simulink model "pendulumExample2"  (Simulink 7.3)
settings: Solver=ode3  StartTime=0.0  StopTime=tof  FixedStep=0.01  RelTol=1e-3
InitFcn:
  | initPendulum2
StopFcn:
  | plotlab
values from neighbouring files (symbols this model uses):
  Arm = [0 1;-wn^2 -2*ksi*wn]    [init.m]    (also in initPendulum2.m)
  B = [0 1]'    [init.m]    (also in initPendulum2.m = [0 0 ; 0 1])
  Brm = [0 wn^2]'    [init.m]    (also in initPendulum2.m)
  epsilon = 0.08    [init.m]    (also in initPendulum2.m)
  GammaW = 3.5    [init.m]    (also in initPendulum2.m)
  K = [1.5 0;0 1.3]    [init.m]    (also in initPendulum2.m)
  nofbasis = 3    [initPendulum2.m]
  nofstates = 2    [initPendulum2.m]
  P = lyap(A',Q)    [init.m]    (also in initPendulum2.m)
  pMax = 10    [initPendulum2.m]
  W0 = [2 -0.5 1]'    [init.m]    (also in initPendulum2.m = [2 -0.5 1 ; 0 0 0]')
  x0 = [1 1]'    [init.m]    (also in initPendulum2.m)
libraries: dspbuff3 x2, simulink x1, dspmtrx3 x1
settings Model: Creator=Alp  LastModifiedBy=alp.marangoz

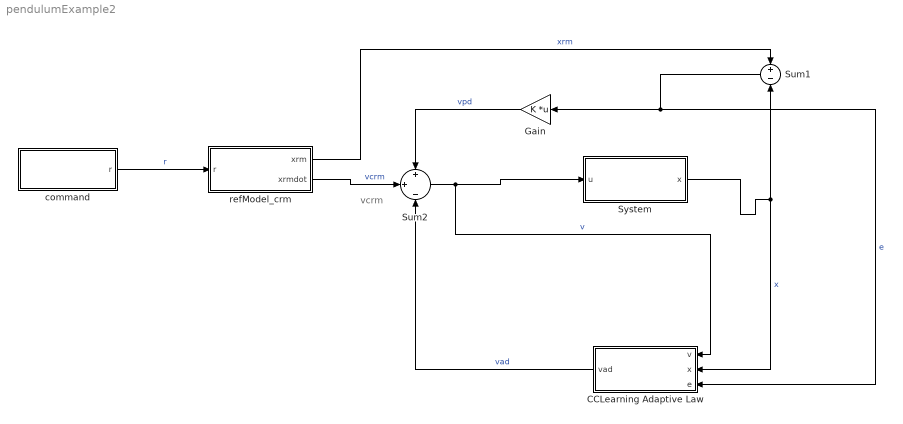
== system pendulumExample2 ==
  note: vcrm
  CCLearning Adaptive Law : Subsystem  TreatAsAtomicUnit=on
  Gain : Gain  Gain=K  Multiplication=Matrix(K*u)  ParameterDataType=fixdt(1, 16)  ParameterScaling=2^0  OutDataType=fixdt(1, 16)  OutScaling=2^0
  Sum1 : Sum  Inputs=+|-  OutDataType=fixdt(1, 16)  OutScaling=2^0
  Sum2 : Sum  Inputs=+|+|-  OutDataType=fixdt(1, 16)  OutScaling=2^0
  System : Subsystem  TreatAsAtomicUnit=on
  command : Subsystem
  refModel_crm : Subsystem  TreatAsAtomicUnit=on
  wires:
  command/1(r) -> refModel_crm/1(r)  "r"
  refModel_crm/1(xrm) -> Sum1/1  "xrm"
  Sum1/1 -> Gain/1, CCLearning Adaptive Law/3(e)  "e"
  Gain/1 -> Sum2/1  "vpd"
  refModel_crm/2(xrmdot) -> Sum2/2  "vcrm"
  Sum2/1 -> System/1(u), CCLearning Adaptive Law/1(v)  "v"
  CCLearning Adaptive Law/1(vad) -> Sum2/3  "vad"
  System/1(x) -> Sum1/2, CCLearning Adaptive Law/2(x)  "x"

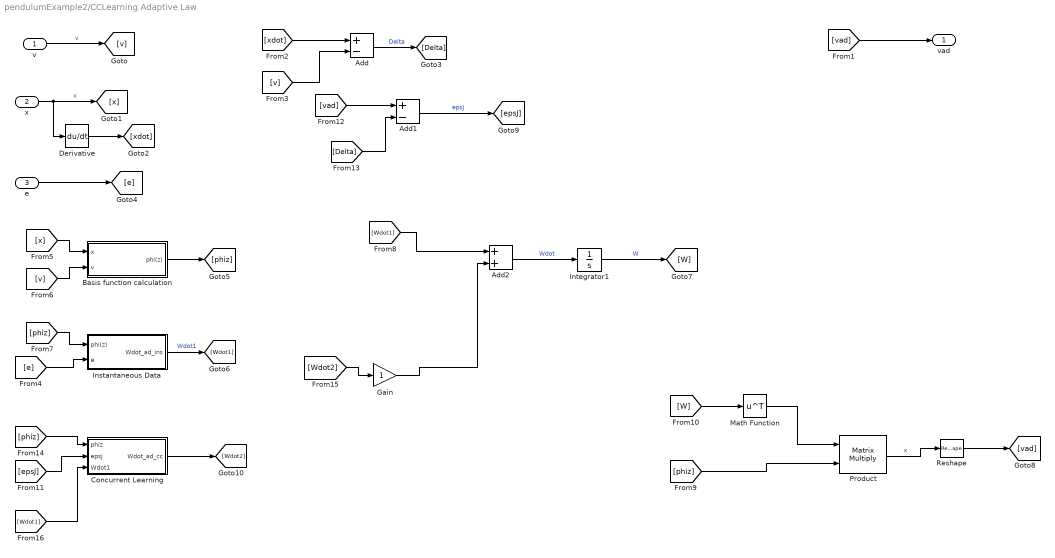
== system pendulumExample2/CCLearning Adaptive Law ==
  v : Inport  OutDataType=fixdt(1, 16)  OutScaling=2^0
  x : Inport  Port=2  OutDataType=fixdt(1, 16)  OutScaling=2^0
  e : Inport  Port=3  OutDataType=fixdt(1, 16)  OutScaling=2^0
  Add : Sum  Inputs=+-  OutDataType=fixdt(1, 16)  OutScaling=2^-10
  Add1 : Sum  Inputs=+-  OutDataType=fixdt(1, 16)  OutScaling=2^-10
  Add2 : Sum  OutDataType=fixdt(1, 16)  OutScaling=2^-10
  Basis function calculation : Subsystem  TreatAsAtomicUnit=on
  Concurrent Learning : Subsystem  TreatAsAtomicUnit=on
  Derivative : Derivative
  Gain : Gain  ParameterDataType=fixdt(1, 16)  ParameterScaling=2^0  OutDataType=fixdt(1, 16)  OutScaling=2^0
  Instantaneous Data : Subsystem  TreatAsAtomicUnit=on
  Integrator1 : Integrator  InitialCondition=W0
  Math Function : Math  Operator=transpose  OutDataType=fixdt(1, 16)  OutScaling=2^0  SaturateOnIntegerOverflow=on
  Product : Product  Multiplication=Matrix(*)  OutDataType=fixdt(1, 16)  OutScaling=2^0  RndMeth=Zero
  Reshape : Reshape  OutputDimensionality=Column vector (2-D)
  vad : Outport  OutDataType=fixdt(1, 16)  OutScaling=2^0
  wires:
  v/1 -> [v]  "v"
  [vad] -> vad/1
  x/1 -> [x], Derivative/1  "x"
  Derivative/1 -> [xdot]
  [xdot] -> Add/1
  [v] -> Add/2
  Add/1 -> [Delta]  "Delta"
  e/1 -> [e]
  [e] -> Instantaneous Data/2(e)
  [x] -> Basis function calculation/1(x)
  [v] -> Basis function calculation/2(v)
  Basis function calculation/1(phi(z)) -> [phiz]
  [phiz] -> Instantaneous Data/1(phi(z))
  Instantaneous Data/1(Wdot_ad_ins) -> [Wdot1]  "Wdot1"
  Integrator1/1 -> [W]  "W"
  [W] -> Math Function/1
  Math Function/1 -> Product/1
  [phiz] -> Product/2
  Product/1 -> Reshape/1  "x"
  Reshape/1 -> [vad]
  [vad] -> Add1/1
  [Delta] -> Add1/2
  Add1/1 -> [epsJ]  "epsJ"
  [phiz] -> Concurrent Learning/1(phiz)
  Concurrent Learning/1(Wdot_ad_cc) -> [Wdot2]
  [epsJ] -> Concurrent Learning/2(epsj)
  [Wdot1] -> Add2/1
  Add2/1 -> Integrator1/1  "Wdot"
  [Wdot2] -> Gain/1
  [Wdot1] -> Concurrent Learning/3(Wdot1)
  Gain/1 -> Add2/2

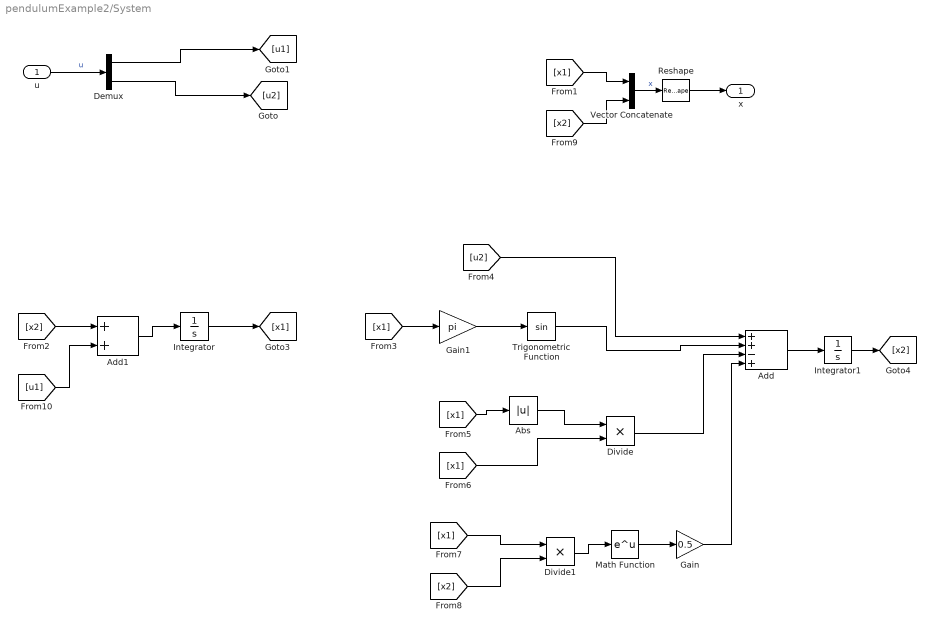
== system pendulumExample2/System ==
  u : Inport  OutDataType=fixdt(1, 16)  OutScaling=2^0
  Abs : Abs  OutDataType=fixdt(1, 16)  OutScaling=2^0
  Add : Sum  Inputs=++-+  OutDataType=fixdt(1, 16)  OutScaling=2^-10
  Add1 : Sum  OutDataType=fixdt(1, 16)  OutScaling=2^-10
  Demux : Demux  Outputs=2
  Divide : Product  Inputs=**  OutDataType=fixdt(1, 16)  OutScaling=2^-10
  Divide1 : Product  Inputs=**  OutDataType=fixdt(1, 16)  OutScaling=2^-10
  Gain : Gain  Gain=0.5  ParameterDataType=fixdt(1, 16)  ParameterScaling=2^0  OutDataType=fixdt(1, 16)  OutScaling=2^0
  Gain1 : Gain  Gain=pi  ParameterDataType=fixdt(1, 16)  ParameterScaling=2^0  OutDataType=fixdt(1, 16)  OutScaling=2^0
  Integrator : Integrator  InitialCondition=x0(1,1)
  Integrator1 : Integrator  InitialCondition=x0(2,1)
  Math Function : Math  OutDataType=fixdt(1, 16)  OutScaling=2^0  SaturateOnIntegerOverflow=on
  Reshape : Reshape  OutputDimensionality=Column vector (2-D)
  Trigonometric Function : Trigonometry
  Vector Concatenate : Concatenate  Mode=Vector
  x : Outport  OutDataType=fixdt(1, 16)  OutScaling=2^0
  wires:
  Integrator/1 -> [x1]
  [x1] -> Gain1/1
  [x1] -> Abs/1
  Abs/1 -> Divide/1
  [x1] -> Divide/2
  [x1] -> Divide1/1
  [x2] -> Divide1/2
  Divide1/1 -> Math Function/1
  Math Function/1 -> Gain/1
  [u2] -> Add/1
  Trigonometric Function/1 -> Add/2
  Divide/1 -> Add/3
  Gain/1 -> Add/4
  Add/1 -> Integrator1/1
  Integrator1/1 -> [x2]
  [x1] -> Vector Concatenate/1
  [x2] -> Vector Concatenate/2
  Vector Concatenate/1 -> Reshape/1  "x"
  Reshape/1 -> x/1
  u/1 -> Demux/1  "u"
  Demux/1 -> [u1]
  Demux/2 -> [u2]
  Gain1/1 -> Trigonometric Function/1
  [x2] -> Add1/1
  Add1/1 -> Integrator/1
  [u1] -> Add1/2

== system pendulumExample2/command ==
  Demux : Demux  Outputs=2
  From Workspace : FromWorkspace  VariableName=rData  OutputAfterFinalValue=Setting to zero
  Reshape : Reshape  OutputDimensionality=Column vector (2-D)
  Terminator1 : Terminator
  r : Outport
  wires:
  From Workspace/1 -> Reshape/1  "r"
  Reshape/1 -> Demux/1
  Demux/1 -> Terminator1/1  "r1"
  Demux/2 -> r/1  "r2"

== system pendulumExample2/refModel_crm ==
  r : Inport  OutDataType=fixdt(1, 16)  OutScaling=2^0
  Add1 : Sum  OutDataType=fixdt(1, 16)  OutScaling=2^-10
  Gain1 : Gain  Gain=Arm  Multiplication=Matrix(K*u)  ParameterDataType=fixdt(1, 16)  ParameterScaling=2^0  OutDataType=fixdt(1, 16)  OutScaling=2^0
  Gain2 : Gain  Gain=Brm  Multiplication=Matrix(K*u)  ParameterDataType=fixdt(1, 16)  ParameterScaling=2^0  OutDataType=fixdt(1, 16)  OutScaling=2^0
  Integrator : Integrator  InitialCondition=x0
  Reshape : Reshape  OutputDimensionality=Column vector (2-D)
  xrm : Outport  OutDataType=fixdt(1, 16)  OutScaling=2^0
  xrmdot : Outport  Port=2  OutDataType=fixdt(1, 16)  OutScaling=2^0
  wires:
  [x] -> Gain1/1
  r/1 -> [u]  "r"
  [u] -> Gain2/1
  Gain1/1 -> Add1/1
  Gain2/1 -> Add1/2
  Add1/1 -> Reshape/1  "xrmdot"
  Integrator/1 -> xrm/1, [x]  "xrm"
  Reshape/1 -> Integrator/1, xrmdot/1

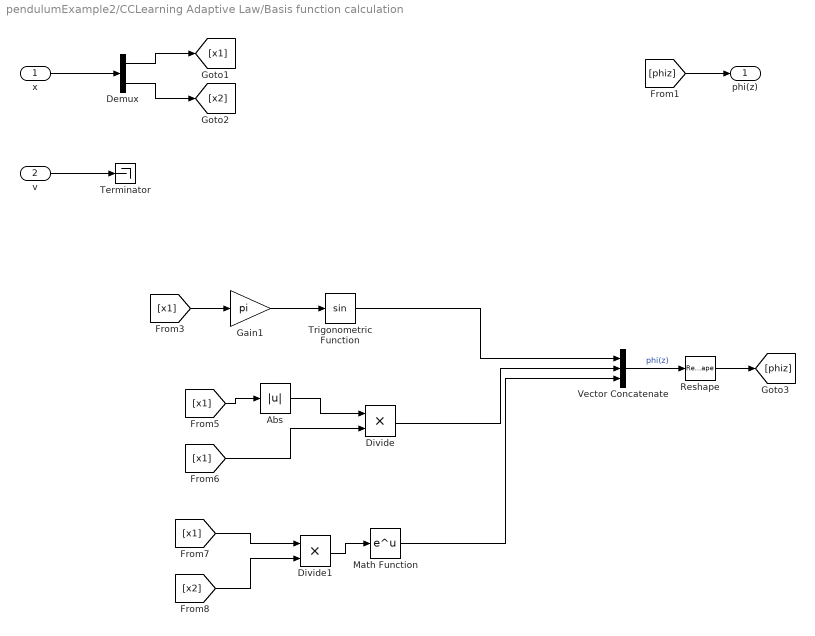
== system pendulumExample2/CCLearning Adaptive Law/Basis function calculation ==
  x : Inport  OutDataType=fixdt(1, 16)  OutScaling=2^0
  v : Inport  Port=2  OutDataType=fixdt(1, 16)  OutScaling=2^0
  Abs : Abs  OutDataType=fixdt(1, 16)  OutScaling=2^0
  Demux : Demux  Outputs=2
  Divide : Product  Inputs=**  OutDataType=fixdt(1, 16)  OutScaling=2^-10
  Divide1 : Product  Inputs=**  OutDataType=fixdt(1, 16)  OutScaling=2^-10
  Gain1 : Gain  Gain=pi  ParameterDataType=fixdt(1, 16)  ParameterScaling=2^0  OutDataType=fixdt(1, 16)  OutScaling=2^0
  Math Function : Math  OutDataType=fixdt(1, 16)  OutScaling=2^0  SaturateOnIntegerOverflow=on
  Reshape : Reshape  OutputDimensionality=Column vector (2-D)
  Terminator : Terminator
  Trigonometric Function : Trigonometry
  Vector Concatenate : Concatenate  NumInputs=3  Mode=Vector
  phi(z) : Outport  OutDataType=fixdt(1, 16)  OutScaling=2^0
  wires:
  x/1 -> Demux/1
  v/1 -> Terminator/1
  [phiz] -> phi(z)/1
  [x1] -> Gain1/1
  [x1] -> Abs/1
  Abs/1 -> Divide/1
  [x1] -> Divide/2
  [x1] -> Divide1/1
  [x2] -> Divide1/2
  Divide1/1 -> Math Function/1
  Gain1/1 -> Trigonometric Function/1
  Demux/1 -> [x1]
  Demux/2 -> [x2]
  Vector Concatenate/1 -> Reshape/1  "phi(z)"
  Reshape/1 -> [phiz]
  Trigonometric Function/1 -> Vector Concatenate/1
  Divide/1 -> Vector Concatenate/2
  Math Function/1 -> Vector Concatenate/3

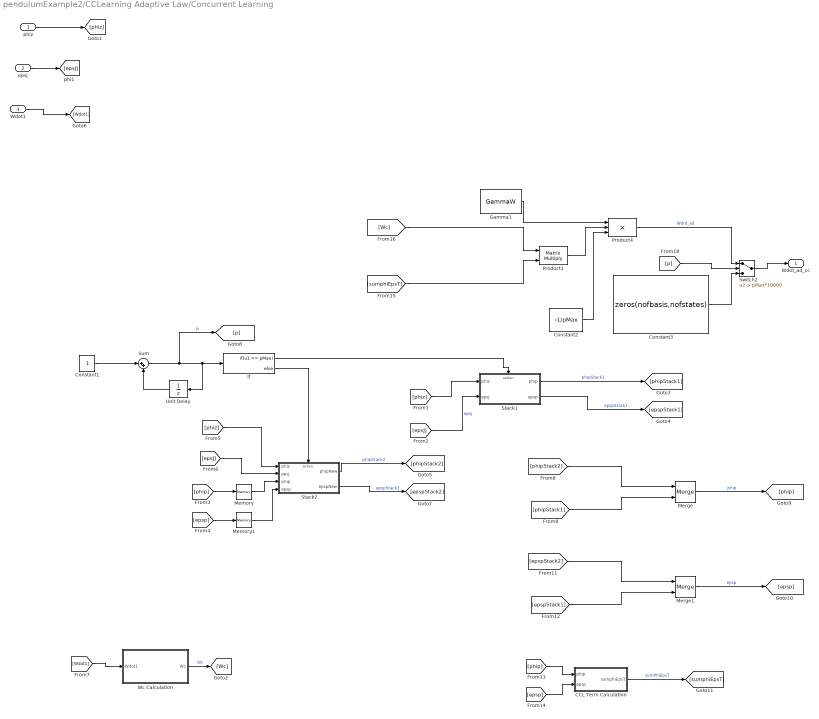
== system pendulumExample2/CCLearning Adaptive Law/Concurrent Learning ==
  phiz : Inport  OutDataType=fixdt(1, 16)  OutScaling=2^0
  epsj : Inport  Port=2  OutDataType=fixdt(1, 16)  OutScaling=2^0
  Wdot1 : Inport  Port=3
  CCL Term Calculation : Subsystem  TreatAsAtomicUnit=on
  Constant1 : Constant  OutDataType=fixdt(1, 16)  OutScaling=2^0  SampleTime=-1
  Constant2 : Constant  Value=-1/pMax  OutDataType=fixdt(1, 16)  OutScaling=2^0
  Constant3 : Constant  Value=zeros(nofbasis,nofstates)  OutDataType=fixdt(1, 16)  OutScaling=2^0  SampleTime=-1
  Gamma1 : Constant  Value=GammaW  VectorParams1D=off  OutDataType=fixdt(1, 16)  OutScaling=2^0
  If : If  IfExpression=u1 <= pMax
  Memory : Memory  X0=zeros(nofbasis,pMax)  InheritSampleTime=on  LinearizeMemory=on  LinearizeAsDelay=on
  Memory1 : Memory  X0=zeros(nofstates,pMax)  InheritSampleTime=on  LinearizeMemory=on  LinearizeAsDelay=on
  Merge : Merge
  Merge1 : Merge
  Product1 : Product  Multiplication=Matrix(*)  OutDataType=fixdt(1, 16)  OutScaling=2^0  RndMeth=Zero
  Product4 : Product  Inputs=3  OutDataType=fixdt(1, 16)  OutScaling=2^0  RndMeth=Zero
  Stack1 : Subsystem  TreatAsAtomicUnit=on
  Stack2 : Subsystem  TreatAsAtomicUnit=on
  Sum : Sum  Inputs=|++  OutDataType=fixdt(1, 16)  OutScaling=2^0
  Switch2 : Switch  Criteria=u2 > Threshold  Threshold=pMax*10000  OutDataType=fixdt(1, 16)  OutScaling=2^0
  Unit Delay : UnitDelay  SampleTime=-1
  Wc Calculation : Subsystem
  Wdot_ad_cc : Outport  OutDataType=fixdt(1, 16)  OutScaling=2^0
  wires:
  phiz/1 -> [phiz]
  epsj/1 -> [epsJ]
  Wdot1/1 -> [Wdot1]
  Gamma1/1 -> Product4/1
  Constant1/1 -> Sum/1
  Sum/1 -> Unit Delay/1, If/1, [p]  "p"
  Unit Delay/1 -> Sum/2
  If/1 -> Stack1/Action
  [epsJ] -> Stack1/2(epsj)  "epsj"
  Stack1/1(phip) -> [phipStack1]  "phipStack1"
  Stack1/2(epsp) -> [epspStack1]  "epspStack1"
  [phiz] -> Stack2/1(phiz)
  [epsJ] -> Stack2/2(epsj)
  If/2 -> Stack2/Action
  [phip] -> Memory/1
  Memory/1 -> Stack2/3(phip)
  [epsp] -> Memory1/1
  Memory1/1 -> Stack2/4(epsp)
  Stack2/1(phipNew) -> [phipStack2]  "phipStack2"
  Stack2/2(epspNew) -> [epspStack2]  "epspStack2"
  [phiz] -> Stack1/1(phiz)
  Merge/1 -> [phip]  "phip"
  Merge1/1 -> [epsp]  "epsp"
  [phip] -> CCL Term Calculation/1(phip)
  [epsp] -> CCL Term Calculation/2(epsp)
  CCL Term Calculation/1(sumphiEpsT) -> [sumphiEpsT]  "sumPhiEpsT"
  Constant2/1 -> Product4/3
  [Wc] -> Product1/1
  [sumphiEpsT] -> Product1/2
  Product1/1 -> Product4/2
  [p] -> Switch2/2
  Constant3/1 -> Switch2/3
  Product4/1 -> Switch2/1  "Wdot_ad"
  Switch2/1 -> Wdot_ad_cc/1
  [phipStack2] -> Merge/1
  [phipStack1] -> Merge/2
  [epspStack2] -> Merge1/1
  [epspStack1] -> Merge1/2
  [Wdot1] -> Wc Calculation/1(Wdot1)
  Wc Calculation/1(Wc) -> [Wc]  "Wc"

== system pendulumExample2/CCLearning Adaptive Law/Instantaneous Data ==
  phi(z) : Inport  OutDataType=fixdt(1, 16)  OutScaling=2^0
  e : Inport  Port=2  OutDataType=fixdt(1, 16)  OutScaling=2^0
  Gain : Gain  Gain=-1  ParameterDataType=fixdt(1, 16)  ParameterScaling=2^0  OutDataType=fixdt(1, 16)  OutScaling=2^0
  Gamma : Constant  Value=GammaW  VectorParams1D=off  OutDataType=fixdt(1, 16)  OutScaling=2^0
  P : Constant  Value=P  VectorParams1D=off  OutDataType=fixdt(1, 16)  OutScaling=2^0
  Product1 : Product  Multiplication=Matrix(*)  OutDataType=fixdt(1, 16)  OutScaling=2^0  RndMeth=Zero
  Product2 : Product  OutDataType=fixdt(1, 16)  OutScaling=2^0  RndMeth=Zero
  Product3 : Product  Multiplication=Matrix(*)  OutDataType=fixdt(1, 16)  OutScaling=2^0  RndMeth=Zero
  Product5 : Product  Multiplication=Matrix(*)  OutDataType=fixdt(1, 16)  OutScaling=2^0  RndMeth=Zero
  Transpose2 : dspmtrx3/Transpose  SystemSampleTime=-1  Hermitian=off  overflowFlag=off
  b : Constant  Value=B  VectorParams1D=off  OutDataType=fixdt(1, 16)  OutScaling=2^0
  Wdot_ad_ins : Outport  OutDataType=fixdt(1, 16)  OutScaling=2^0
  wires:
  P/1 -> Product5/1
  b/1 -> Product5/2
  e/1 -> Transpose2/1
  Transpose2/1 -> Product1/1
  Product5/1 -> Product1/2
  phi(z)/1 -> Product3/1
  Product1/1 -> Product3/2
  Gamma/1 -> Product2/1
  Product3/1 -> Product2/2
  Product2/1 -> Gain/1
  Gain/1 -> Wdot_ad_ins/1

== system pendulumExample2/CCLearning Adaptive Law/Concurrent Learning/CCL Term Calculation ==
  phip : Inport  OutDataType=fixdt(1, 16)  OutScaling=2^0
  epsp : Inport  Port=2  OutDataType=fixdt(1, 16)  OutScaling=2^0
  For Iterator Subsystem : Subsystem  TreatAsAtomicUnit=on
  Memory2 : Memory  X0=zeros(size(W0))  InheritSampleTime=on  LinearizeMemory=on  LinearizeAsDelay=on
  sumphiEpsT : Outport  OutDataType=fixdt(1, 16)  OutScaling=2^0
  wires:
  epsp/1 -> [epsp]
  phip/1 -> [phip]
  [phip] -> For Iterator Subsystem/1(phip)
  [epsp] -> For Iterator Subsystem/2(epsp)
  For Iterator Subsystem/2(forSumphiEpsTnext) -> Memory2/1
  Memory2/1 -> For Iterator Subsystem/3(forSumphiEpsT)
  For Iterator Subsystem/1(sumphiEpsT) -> [sumphiEpsT]
  [sumphiEpsT] -> sumphiEpsT/1

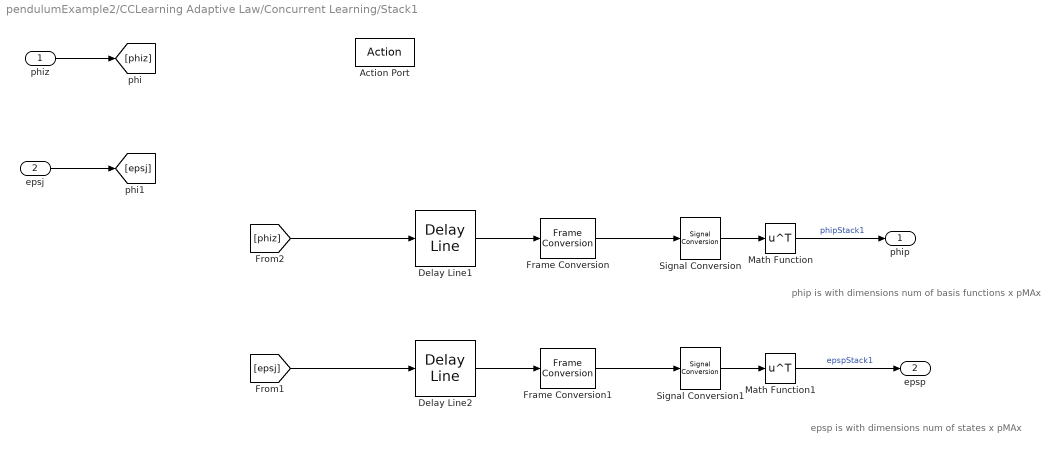
== system pendulumExample2/CCLearning Adaptive Law/Concurrent Learning/Stack1 ==
  note: phip is with dimensions num of basis functions x pMAx
  note: epsp is with dimensions num of states x pMAx
  phiz : Inport  OutDataType=fixdt(1, 16)  OutScaling=2^0
  epsj : Inport  Port=2  OutDataType=fixdt(1, 16)  OutScaling=2^0
  Action Port : ActionPort  ActionType=then
  Delay Line1 : dspbuff3/Delay Line  siz=pMax  ic=0  directfeed=on  enable_output=off  hold_output=off
  Delay Line2 : dspbuff3/Delay Line  siz=pMax  ic=0  directfeed=on  enable_output=off  hold_output=off
  Frame Conversion : FrameConversion  OutFrame=Sample-based
  Frame Conversion1 : FrameConversion  OutFrame=Sample-based
  Math Function : Math  Operator=transpose  OutDataType=fixdt(1, 16)  OutScaling=2^0  SaturateOnIntegerOverflow=on
  Math Function1 : Math  Operator=transpose  OutDataType=fixdt(1, 16)  OutScaling=2^0  SaturateOnIntegerOverflow=on
  Signal Conversion : SignalConversion  ConversionOutput=Contiguous copy
  Signal Conversion1 : SignalConversion  ConversionOutput=Contiguous copy
  phip : Outport  OutDataType=fixdt(1, 16)  OutScaling=2^0
  epsp : Outport  Port=2  OutDataType=fixdt(1, 16)  OutScaling=2^0
  wires:
  phiz/1 -> [phiz]
  Delay Line1/1 -> Frame Conversion/1
  epsj/1 -> [epsj]
  Frame Conversion/1 -> Signal Conversion/1
  [phiz] -> Delay Line1/1
  Delay Line2/1 -> Frame Conversion1/1
  Frame Conversion1/1 -> Signal Conversion1/1
  [epsj] -> Delay Line2/1
  Signal Conversion/1 -> Math Function/1
  Signal Conversion1/1 -> Math Function1/1
  Math Function/1 -> phip/1  "phipStack1"
  Math Function1/1 -> epsp/1  "epspStack1"

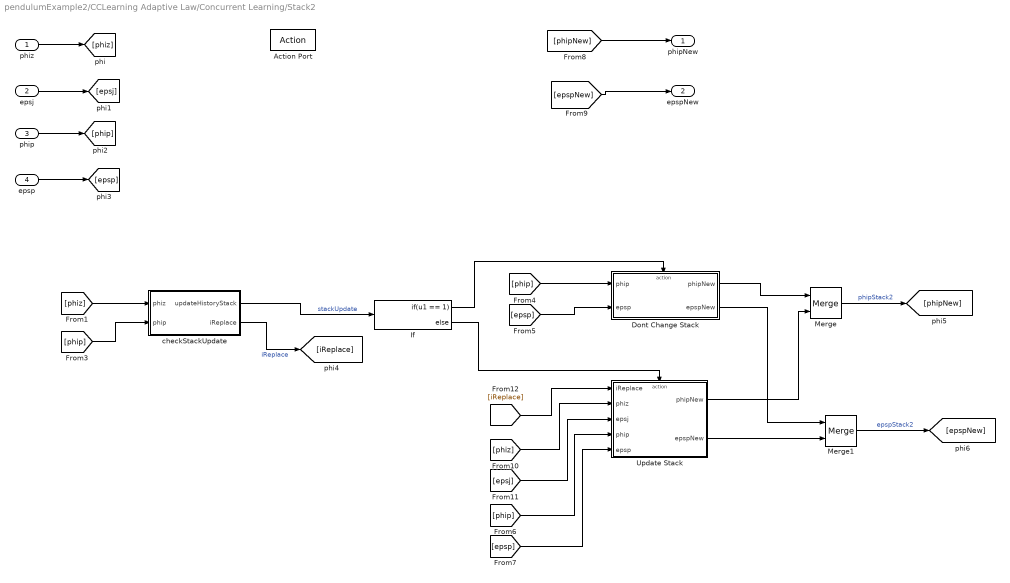
== system pendulumExample2/CCLearning Adaptive Law/Concurrent Learning/Stack2 ==
  phiz : Inport  OutDataType=fixdt(1, 16)  OutScaling=2^0
  epsj : Inport  Port=2  OutDataType=fixdt(1, 16)  OutScaling=2^0
  phip : Inport  Port=3  OutDataType=fixdt(1, 16)  OutScaling=2^0
  epsp : Inport  Port=4  OutDataType=fixdt(1, 16)  OutScaling=2^0
  Action Port : ActionPort  ActionType=else
  Dont Change Stack : Subsystem  TreatAsAtomicUnit=on
  If : If  IfExpression=u1 == 1
  Merge : Merge
  Merge1 : Merge
  Update Stack : Subsystem  TreatAsAtomicUnit=on
  checkStackUpdate : Subsystem  TreatAsAtomicUnit=on
  phipNew : Outport  OutDataType=fixdt(1, 16)  OutScaling=2^0
  epspNew : Outport  Port=2  OutDataType=fixdt(1, 16)  OutScaling=2^0
  wires:
  epsj/1 -> [epsj]
  phiz/1 -> [phiz]
  epsp/1 -> [epsp]
  phip/1 -> [phip]
  [phipNew] -> phipNew/1
  [epspNew] -> epspNew/1
  If/1 -> Dont Change Stack/Action
  If/2 -> Update Stack/Action
  [iReplace] -> Update Stack/1(iReplace)
  [phiz] -> Update Stack/2(phiz)
  [epsj] -> Update Stack/3(epsj)
  [phip] -> Update Stack/4(phip)
  [epsp] -> Update Stack/5(epsp)
  Dont Change Stack/1(phipNew) -> Merge/1
  Dont Change Stack/2(epspNew) -> Merge1/1
  Update Stack/1(phipNew) -> Merge/2
  Update Stack/2(epspNew) -> Merge1/2
  [phip] -> Dont Change Stack/1(phip)
  [epsp] -> Dont Change Stack/2(epsp)
  Merge/1 -> [phipNew]  "phipStack2"
  Merge1/1 -> [epspNew]  "epspStack2"
  [phiz] -> checkStackUpdate/1(phiz)
  [phip] -> checkStackUpdate/2(phip)
  checkStackUpdate/1(updateHistoryStack) -> If/1  "stackUpdate"
  checkStackUpdate/2(iReplace) -> [iReplace]  "iReplace"

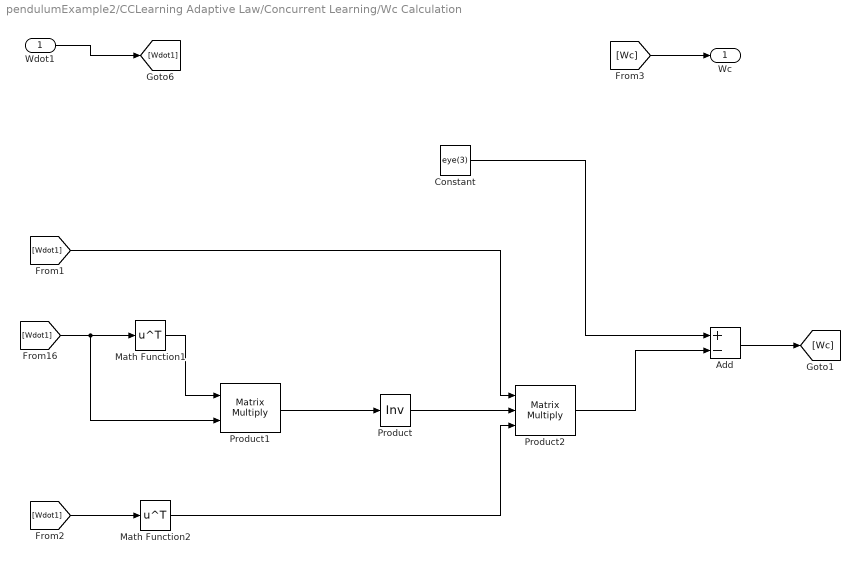
== system pendulumExample2/CCLearning Adaptive Law/Concurrent Learning/Wc Calculation ==
  Wdot1 : Inport
  Add : Sum  Inputs=+-  OutDataType=fixdt(1, 16)  OutScaling=2^-10
  Constant : Constant  Value=eye(3)  OutDataType=fixdt(1, 16)  OutScaling=2^0
  Math Function1 : Math  Operator=transpose  OutDataType=fixdt(1, 16)  OutScaling=2^0  SaturateOnIntegerOverflow=on
  Math Function2 : Math  Operator=transpose  OutDataType=fixdt(1, 16)  OutScaling=2^0  SaturateOnIntegerOverflow=on
  Product : Product  Inputs=/  Multiplication=Matrix(*)  OutDataType=fixdt(1, 16)  OutScaling=2^0  RndMeth=Zero
  Product1 : Product  Multiplication=Matrix(*)  OutDataType=fixdt(1, 16)  OutScaling=2^0  RndMeth=Zero
  Product2 : Product  Inputs=***  Multiplication=Matrix(*)  OutDataType=fixdt(1, 16)  OutScaling=2^0  RndMeth=Zero
  Wc : Outport
  wires:
  [Wdot1] -> Math Function1/1, Product1/2
  Math Function1/1 -> Product1/1
  Product1/1 -> Product/1
  Wdot1/1 -> [Wdot1]
  [Wdot1] -> Math Function2/1
  [Wdot1] -> Product2/1
  Product/1 -> Product2/2
  Math Function2/1 -> Product2/3
  Constant/1 -> Add/1
  Add/1 -> [Wc]
  [Wc] -> Wc/1
  Product2/1 -> Add/2

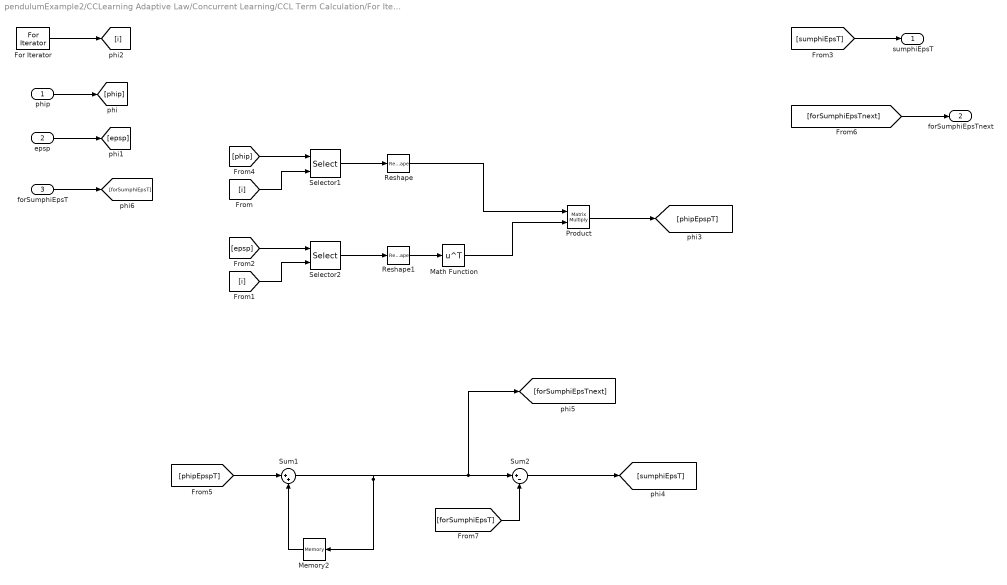
== system pendulumExample2/CCLearning Adaptive Law/Concurrent Learning/CCL Term Calculation/For Iterator Subsystem ==
  phip : Inport  OutDataType=fixdt(1, 16)  OutScaling=2^0
  epsp : Inport  Port=2  OutDataType=fixdt(1, 16)  OutScaling=2^0
  forSumphiEpsT : Inport  Port=3  OutDataType=fixdt(1, 16)  OutScaling=2^0
  For Iterator : ForIterator  IterationLimit=pMax
  Math Function : Math  Operator=transpose  OutDataType=fixdt(1, 16)  OutScaling=2^0  SaturateOnIntegerOverflow=on
  Memory2 : Memory  X0=zeros(size(W0))  InheritSampleTime=on  LinearizeMemory=on  LinearizeAsDelay=on
  Product : Product  Multiplication=Matrix(*)  OutDataType=fixdt(1, 16)  OutScaling=2^0  RndMeth=Zero
  Reshape : Reshape  OutputDimensionality=Column vector (2-D)
  Reshape1 : Reshape  OutputDimensionality=Column vector (2-D)
  Selector1 : Selector  NumberOfDimensions=2  InputPortWidth=3  IndexOptions=Select all,Index vector (port)  Indices=[1 2 3],1  OutputSizes=1,1
  Selector2 : Selector  NumberOfDimensions=2  InputPortWidth=3  IndexOptions=Select all,Index vector (port)  Indices=[1 2 3],1  OutputSizes=1,1
  Sum1 : Sum  Inputs=|++  OutDataType=fixdt(1, 16)  OutScaling=2^0
  Sum2 : Sum  Inputs=|+-  OutDataType=fixdt(1, 16)  OutScaling=2^0
  sumphiEpsT : Outport  OutDataType=fixdt(1, 16)  OutScaling=2^0
  forSumphiEpsTnext : Outport  Port=2  OutDataType=fixdt(1, 16)  OutScaling=2^0
  wires:
  epsp/1 -> [epsp]
  phip/1 -> [phip]
  For Iterator/1 -> [i]
  [sumphiEpsT] -> sumphiEpsT/1
  [phip] -> Selector1/1
  [i] -> Selector1/2
  Selector1/1 -> Reshape/1
  [epsp] -> Selector2/1
  [i] -> Selector2/2
  Selector2/1 -> Reshape1/1
  Reshape1/1 -> Math Function/1
  Reshape/1 -> Product/1
  Math Function/1 -> Product/2
  Product/1 -> [phipEpspT]
  Sum1/1 -> Memory2/1, Sum2/1, [forSumphiEpsTnext]
  [phipEpspT] -> Sum1/1
  Memory2/1 -> Sum1/2
  Sum2/1 -> [sumphiEpsT]
  [forSumphiEpsT] -> Sum2/2
  forSumphiEpsT/1 -> [forSumphiEpsT]
  [forSumphiEpsTnext] -> forSumphiEpsTnext/1

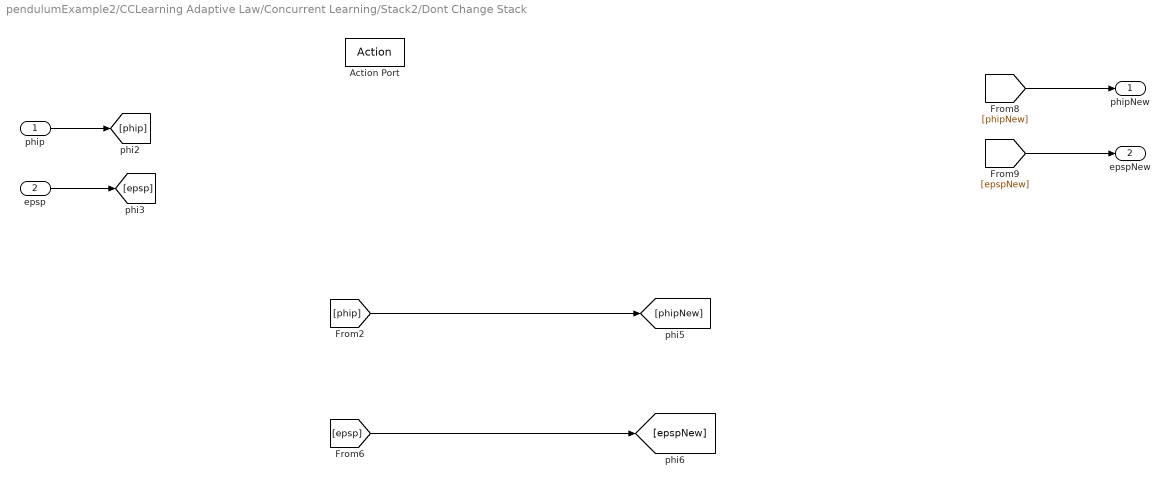
== system pendulumExample2/CCLearning Adaptive Law/Concurrent Learning/Stack2/Dont Change Stack ==
  phip : Inport  OutDataType=fixdt(1, 16)  OutScaling=2^0
  epsp : Inport  Port=2  OutDataType=fixdt(1, 16)  OutScaling=2^0
  Action Port : ActionPort  ActionType=then
  phipNew : Outport  OutDataType=fixdt(1, 16)  OutScaling=2^0
  epspNew : Outport  Port=2  OutDataType=fixdt(1, 16)  OutScaling=2^0
  wires:
  epsp/1 -> [epsp]
  phip/1 -> [phip]
  [phipNew] -> phipNew/1
  [epspNew] -> epspNew/1
  [epsp] -> [epspNew]
  [phip] -> [phipNew]

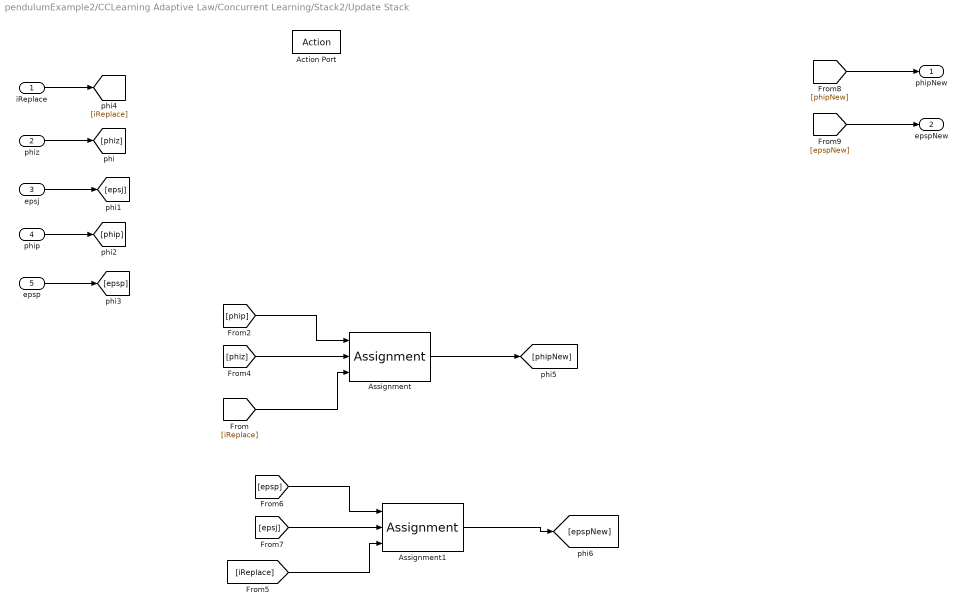
== system pendulumExample2/CCLearning Adaptive Law/Concurrent Learning/Stack2/Update Stack ==
  iReplace : Inport  OutDataType=fixdt(1, 16)  OutScaling=2^0
  phiz : Inport  Port=2  OutDataType=fixdt(1, 16)  OutScaling=2^0
  epsj : Inport  Port=3  OutDataType=fixdt(1, 16)  OutScaling=2^0
  phip : Inport  Port=4  OutDataType=fixdt(1, 16)  OutScaling=2^0
  epsp : Inport  Port=5  OutDataType=fixdt(1, 16)  OutScaling=2^0
  Action Port : ActionPort  ActionType=else
  Assignment : Assignment  NumberOfDimensions=2  IndexOptions=Assign all,Index vector (port)  Indices=1,1  OutputSizes=1,1
  Assignment1 : Assignment  NumberOfDimensions=2  IndexOptions=Assign all,Index vector (port)  Indices=1,1  OutputSizes=1,1
  phipNew : Outport  OutDataType=fixdt(1, 16)  OutScaling=2^0
  epspNew : Outport  Port=2  OutDataType=fixdt(1, 16)  OutScaling=2^0
  wires:
  [iReplace] -> Assignment/3
  [phip] -> Assignment/1
  Assignment/1 -> [phipNew]
  [iReplace] -> Assignment1/3
  [epsp] -> Assignment1/1
  [epsj] -> Assignment1/2
  Assignment1/1 -> [epspNew]
  [phiz] -> Assignment/2
  epsj/1 -> [epsj]
  phiz/1 -> [phiz]
  epsp/1 -> [epsp]
  phip/1 -> [phip]
  [phipNew] -> phipNew/1
  [epspNew] -> epspNew/1
  iReplace/1 -> [iReplace]

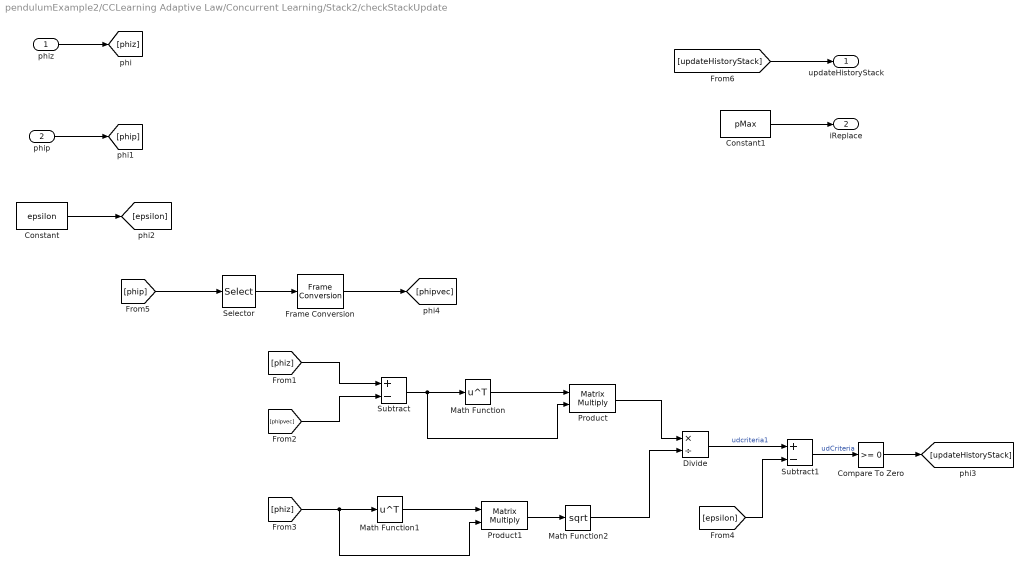
== system pendulumExample2/CCLearning Adaptive Law/Concurrent Learning/Stack2/checkStackUpdate ==
  phiz : Inport  OutDataType=fixdt(1, 16)  OutScaling=2^0
  phip : Inport  Port=2  OutDataType=fixdt(1, 16)  OutScaling=2^0
  Compare To Zero : simulink/Logic and Bit Operations/Compare To Zero  SystemSampleTime=-1  relop=>=  LogicOutDataTypeMode=uint8  ZeroCross=off
  Constant : Constant  Value=epsilon  OutDataType=fixdt(1, 16)  OutScaling=2^0  SampleTime=-1
  Constant1 : Constant  Value=pMax  OutDataType=fixdt(1, 16)  OutScaling=2^0  SampleTime=-1
  Divide : Product  Inputs=*/  OutDataType=fixdt(1, 16)  OutScaling=2^-10
  Frame Conversion : FrameConversion  OutFrame=Sample-based
  Math Function : Math  Operator=transpose  OutDataType=fixdt(1, 16)  OutScaling=2^0  SaturateOnIntegerOverflow=on
  Math Function1 : Math  Operator=transpose  OutDataType=fixdt(1, 16)  OutScaling=2^0  SaturateOnIntegerOverflow=on
  Math Function2 : Math  Operator=sqrt  OutDataType=fixdt(1, 16)  OutScaling=2^0  SaturateOnIntegerOverflow=on
  Product : Product  Multiplication=Matrix(*)  OutDataType=fixdt(1, 16)  OutScaling=2^0  RndMeth=Zero
  Product1 : Product  Multiplication=Matrix(*)  OutDataType=fixdt(1, 16)  OutScaling=2^0  RndMeth=Zero
  Selector : Selector  NumberOfDimensions=2  InputPortWidth=3  IndexOptions=Select all,Index vector (dialog)  Indices=pMax,pMax  OutputSizes=1,1
  Subtract : Sum  Inputs=+-  OutDataType=fixdt(1, 16)  OutScaling=2^-10
  Subtract1 : Sum  Inputs=+-  OutDataType=fixdt(1, 16)  OutScaling=2^-10
  updateHistoryStack : Outport  OutDataType=fixdt(1, 16)  OutScaling=2^0
  iReplace : Outport  Port=2  OutDataType=fixdt(1, 16)  OutScaling=2^0
  wires:
  phip/1 -> [phip]
  phiz/1 -> [phiz]
  Constant1/1 -> iReplace/1
  Constant/1 -> [epsilon]
  [phiz] -> Subtract/1
  [phipvec] -> Subtract/2
  Subtract/1 -> Math Function/1, Product/2
  Math Function/1 -> Product/1
  [phiz] -> Product1/2, Math Function1/1
  Math Function1/1 -> Product1/1
  Product1/1 -> Math Function2/1
  Product/1 -> Divide/1
  Divide/1 -> Subtract1/1  "udcriteria1"
  [epsilon] -> Subtract1/2
  Subtract1/1 -> Compare To Zero/1  "udCriteria"
  Compare To Zero/1 -> [updateHistoryStack]
  Math Function2/1 -> Divide/2
  [phip] -> Selector/1
  Selector/1 -> Frame Conversion/1
  Frame Conversion/1 -> [phipvec]
  [updateHistoryStack] -> updateHistoryStack/1
